simulink model "fre"  (R2021a)
settings: Solver=VariableStepAuto  StartTime=0.0  StopTime=10.0  RelTol=1e-3
settings Model: Creator=HanDong  LastModifiedBy=HanDong

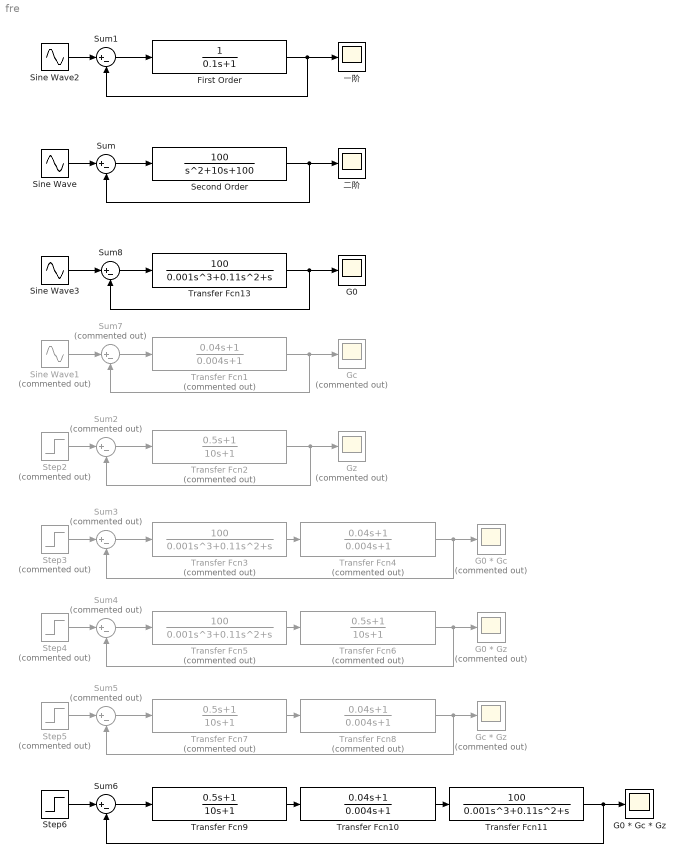
== system fre ==
  First Order : TransferFcn  Denominator=[0.1 1]
  G0 : Scope
  G0 * Gc : Scope  Commented=on
  G0 * Gc * Gz : Scope
  G0 * Gz : Scope  Commented=on
  Gc : Scope  Commented=on
  Gc * Gz : Scope  Commented=on
  Gz : Scope  Commented=on
  Second Order : TransferFcn  Numerator=[100]  Denominator=[1 10 100]
  Sine Wave : Sin  SampleTime=0
  Sine Wave1 : Sin  Commented=on  SampleTime=0
  Sine Wave2 : Sin  SampleTime=0
  Sine Wave3 : Sin  SampleTime=0
  Step{2..5} (4 alike) : Step  Commented=on  Time=0  SampleTime=0
  Step6 : Step  Time=0  SampleTime=0
  Sum{,1,6,8} (4 alike) : Sum  Inputs=|+-
  Sum{2..5,7} (5 alike) : Sum  Commented=on  Inputs=|+-
  Transfer Fcn1 : TransferFcn  Commented=on  Numerator=[0.04 1]  Denominator=[0.004 1]
  Transfer Fcn10 : TransferFcn  Numerator=[0.04 1]  Denominator=[0.004 1]
  Transfer Fcn11 : TransferFcn  Numerator=[100]  Denominator=[0.001 0.11 1 0]
  Transfer Fcn13 : TransferFcn  Numerator=[100]  Denominator=[0.001 0.11 1 0]
  Transfer Fcn2 : TransferFcn  Commented=on  Numerator=[0.5 1]  Denominator=[10 1]
  Transfer Fcn3 : TransferFcn  Commented=on  Numerator=[100]  Denominator=[0.001 0.11 1 0]
  Transfer Fcn4 : TransferFcn  Commented=on  Numerator=[0.04 1]  Denominator=[0.004 1]
  Transfer Fcn5 : TransferFcn  Commented=on  Numerator=[100]  Denominator=[0.001 0.11 1 0]
  Transfer Fcn6 : TransferFcn  Commented=on  Numerator=[0.5 1]  Denominator=[10 1]
  Transfer Fcn7 : TransferFcn  Commented=on  Numerator=[0.5 1]  Denominator=[10 1]
  Transfer Fcn8 : TransferFcn  Commented=on  Numerator=[0.04 1]  Denominator=[0.004 1]
  Transfer Fcn9 : TransferFcn  Numerator=[0.5 1]  Denominator=[10 1]
  一阶 : Scope
  二阶 : Scope
  wires:
  Second Order/1 -> 二阶/1, Sum/2
  Sum/1 -> Second Order/1
  Sine Wave/1 -> Sum/1
  Transfer Fcn2/1 -> Sum2/2, Gz/1
  Sum2/1 -> Transfer Fcn2/1
  Step2/1 -> Sum2/1
  Step3/1 -> Sum3/1
  Sum3/1 -> Transfer Fcn3/1
  Transfer Fcn3/1 -> Transfer Fcn4/1
  Transfer Fcn4/1 -> Sum3/2, G0 * Gc/1
  Transfer Fcn6/1 -> Sum4/2, G0 * Gz/1
  Sum4/1 -> Transfer Fcn5/1
  Step4/1 -> Sum4/1
  Transfer Fcn5/1 -> Transfer Fcn6/1
  Transfer Fcn8/1 -> Sum5/2, Gc * Gz/1
  Sum5/1 -> Transfer Fcn7/1
  Step5/1 -> Sum5/1
  Transfer Fcn7/1 -> Transfer Fcn8/1
  Transfer Fcn9/1 -> Transfer Fcn10/1
  Sum6/1 -> Transfer Fcn9/1
  Step6/1 -> Sum6/1
  Transfer Fcn10/1 -> Transfer Fcn11/1
  Transfer Fcn11/1 -> Sum6/2, G0 * Gc * Gz/1
  Sum7/1 -> Transfer Fcn1/1
  Sine Wave1/1 -> Sum7/1
  Transfer Fcn1/1 -> Gc/1, Sum7/2
  Sine Wave2/1 -> Sum1/1
  Sum1/1 -> First Order/1
  First Order/1 -> Sum1/2, 一阶/1
  Transfer Fcn13/1 -> G0/1, Sum8/2
  Sine Wave3/1 -> Sum8/1
  Sum8/1 -> Transfer Fcn13/1
